simulink model "dq0inverter_DDSRF"  (R2023b)
settings: Solver=VariableStepAuto  StartTime=0.0  StopTime=10.0  RelTol=1e-3
libraries: spsSeriesRLCBranchLib x14, spsGroundLib x10, spsCurrentMeasurementLib x8, spsIGBTDiodeLib x6, slpidlib x4, spsSequenceAnalyzerLib x4, spsabctodq0Lib x4, spsVoltageMeasurementLib x4, spsBreakerLib x3, spsPLLLib x2, spsdq0toabcLib x2, spsDCVoltageSourceLib x1
settings Model: Creator=Jia Yee Wong  LastModifiedBy=Jia Yee Wong

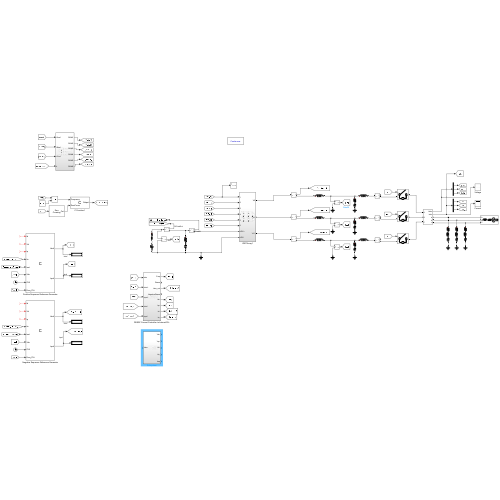
[thumbnail: Simulink's stored preview of the top-level diagram]
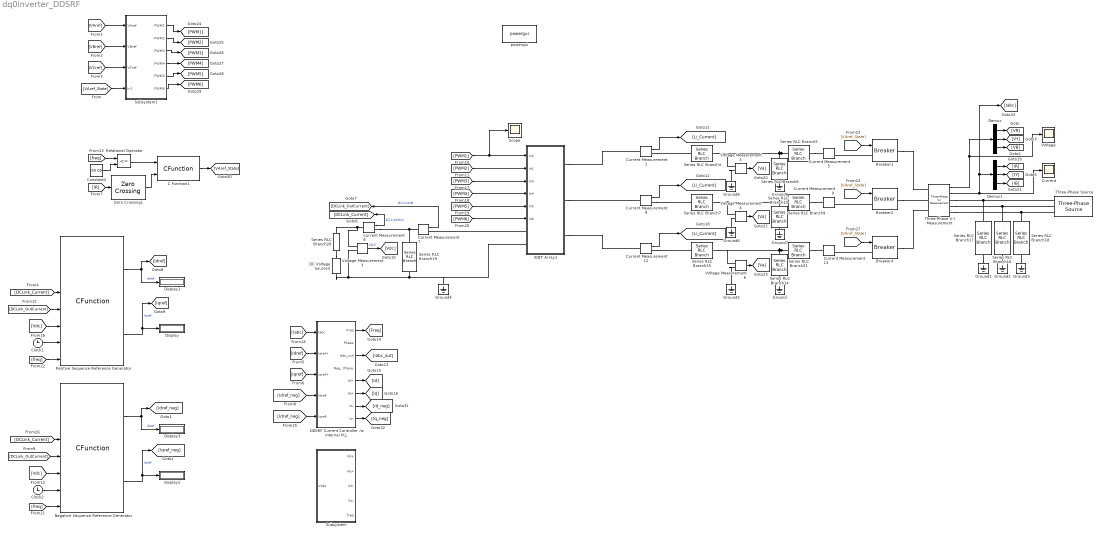
== system dq0inverter_DDSRF ==
  Breaker1 : spsBreakerLib/Breaker  InitialState=0  SwitchingTimes="[1/60  5/60]"  External=on  BreakerResistance=0.00001  SnubberResistance=30  SnubberCapacitance=47e-9  Measurements=None  MoreParameters=on  NoBreakLoop=off
  Breaker2 : spsBreakerLib/Breaker  InitialState=0  SwitchingTimes="[1/60  5/60]"  External=on  BreakerResistance=0.00001  SnubberResistance=30  SnubberCapacitance=47e-9  Measurements=None  MoreParameters=on  NoBreakLoop=off
  Breaker4 : spsBreakerLib/Breaker  InitialState=0  SwitchingTimes="[1/60  5/60]"  External=on  BreakerResistance=0.00001  SnubberResistance=30  SnubberCapacitance=47e-9  Measurements=None  MoreParameters=on  NoBreakLoop=off
  C Function1 : CFunction  OutputCode=|  SampleTime=1/50000
      | if(Frequency == true && ZeroCross == 1){
      |     Output = 1;}
      | else if(Frequency == false){
      |         Output = 0;}
  Clock1 : Clock
  Clock2 : Clock
  Constant4 : Constant  Value=50.05  SampleTime=1/50000
  Current : Scope
  Current Measurement{2,5..9,12..13} (8 alike) : spsCurrentMeasurementLib/Current Measurement  PhasorSimulation=off  OutputType=Complex  PSBequivalent=0
  DC Voltage Source3 : spsDCVoltageSourceLib/DC Voltage Source  Amplitude=400  Measurements=None
  DDSRF Current Controller /w Internal PLL : Subsystem
  Demux : Demux  Outputs=3
  Demux1 : Demux  Outputs=3
  Display{,1..3} (4 alike) : Display
  Ground{,1..9} (10 alike) : spsGroundLib/Ground  LConnTagsString=a
  IGBT Array1 : Subsystem
  Negative Sequence Reference Generator : CFunction  OutputCode=|  StartCode=|  SampleTime=1/50000
      OutputCode=|
      | if(Id!=PreviousId || Iq!=PreviousIq){
      |     if(ReferenceGenTrigger(Freq_PLL)){
      |         Idref=IdrefCalc(CLK,Vd,Iin,Iout, Vdc, Vdc);
      |   //Idref =1;
      |    Iqref=0;
      |    PreviousId=Id;
      |    PreviousIq=Iq;
      |    }
      |   
      | } else { Idref = 0; Iqref = 0;}
      StartCode=|
      | PreviousIq =0;
      | PreviousId =0;
  Positive Sequence Reference Generator : CFunction  OutputCode=|  StartCode=|  SampleTime=1/50000
      OutputCode=|
      | if(Id!=PreviousId || Iq!=PreviousIq){
      |     if(ReferenceGenTrigger(Freq_PLL)){
      |         Idref=IdrefCalc(CLK,Vd,Iin,Iout, Vdc, Vdc);
      |   //Idref =1;
      |    Iqref=0;
      |    PreviousId=Id;
      |    PreviousIq=Iq;
      |    }
      |   
      | } else { Idref = 0; Iqref = 0;}
      StartCode=|
      | PreviousIq =0;
      | PreviousId =0;
  Relational Operator : RelationalOperator  Operator=<=  OutDataTypeStr=boolean  RndMeth=Simplest  InputSameDT=off
  Scope : Scope
  Series RLC Branch10 : spsSeriesRLCBranchLib/Series RLC Branch  LConnTagsString=__new0  RConnTagsString=__new0  BranchType=RC  Resistance=120  Inductance=100e-6  SetiL0=off  InitialCurrent=0  Capacitance=5.526e-6  Setx0=off  InitialVoltage=0  Measurements=None
  Series RLC Branch14 : spsSeriesRLCBranchLib/Series RLC Branch  LConnTagsString=__new0  RConnTagsString=__new0  BranchType=RC  Resistance=120  Inductance=100e-6  SetiL0=off  InitialCurrent=0  Capacitance=5.526e-6  Setx0=off  InitialVoltage=0  Measurements=None
  Series RLC Branch15 : spsSeriesRLCBranchLib/Series RLC Branch  LConnTagsString=__new0  RConnTagsString=__new0  BranchType=L  Resistance=1  Inductance=20.4e-3  SetiL0=off  InitialCurrent=0  Capacitance=1e-6  Setx0=off  InitialVoltage=0  Measurements=None
  Series RLC Branch16 : spsSeriesRLCBranchLib/Series RLC Branch  LConnTagsString=__new0  RConnTagsString=__new0  BranchType=RLC  Resistance=1  Inductance=1e-3  SetiL0=off  InitialCurrent=0  Capacitance=1e-6  Setx0=off  InitialVoltage=0  Measurements=None
  Series RLC Branch17 : spsSeriesRLCBranchLib/Series RLC Branch  LConnTagsString=__new0  RConnTagsString=__new0  BranchType=RLC  Resistance=1  Inductance=1e-3  SetiL0=off  InitialCurrent=0  Capacitance=1e-6  Setx0=off  InitialVoltage=0  Measurements=None
  Series RLC Branch18 : spsSeriesRLCBranchLib/Series RLC Branch  LConnTagsString=__new0  RConnTagsString=__new0  BranchType=RLC  Resistance=1  Inductance=1e-3  SetiL0=off  InitialCurrent=0  Capacitance=1e-6  Setx0=off  InitialVoltage=0  Measurements=None
  Series RLC Branch19 : spsSeriesRLCBranchLib/Series RLC Branch  LConnTagsString=__new0  RConnTagsString=__new0  BranchType=RC  Resistance=1  Inductance=0  SetiL0=off  InitialCurrent=0  Capacitance=47e-3  Setx0=off  InitialVoltage=300  Measurements=None
  Series RLC Branch20 : spsSeriesRLCBranchLib/Series RLC Branch  LConnTagsString=__new0  RConnTagsString=__new0  BranchType=RL  Resistance=100  Inductance=0  SetiL0=off  InitialCurrent=0  Capacitance=1e-6  Setx0=off  InitialVoltage=0  Measurements=None
  Series RLC Branch21 : spsSeriesRLCBranchLib/Series RLC Branch  LConnTagsString=__new0  RConnTagsString=__new0  BranchType=L  Resistance=1  Inductance=148.336e-6  SetiL0=off  InitialCurrent=0  Capacitance=1e-6  Setx0=off  InitialVoltage=0  Measurements=None
  Series RLC Branch4 : spsSeriesRLCBranchLib/Series RLC Branch  LConnTagsString=__new0  RConnTagsString=__new0  BranchType=L  Resistance=1  Inductance=20.4e-3  SetiL0=off  InitialCurrent=0  Capacitance=1e-6  Setx0=off  InitialVoltage=0  Measurements=None
  Series RLC Branch5 : spsSeriesRLCBranchLib/Series RLC Branch  LConnTagsString=__new0  RConnTagsString=__new0  BranchType=L  Resistance=1  Inductance=148.336e-6  SetiL0=off  InitialCurrent=0  Capacitance=1e-6  Setx0=off  InitialVoltage=0  Measurements=None
  Series RLC Branch6 : spsSeriesRLCBranchLib/Series RLC Branch  LConnTagsString=__new0  RConnTagsString=__new0  BranchType=RC  Resistance=120  Inductance=100e-6  SetiL0=off  InitialCurrent=0  Capacitance=5.526e-6  Setx0=off  InitialVoltage=0  Measurements=None
  Series RLC Branch7 : spsSeriesRLCBranchLib/Series RLC Branch  LConnTagsString=__new0  RConnTagsString=__new0  BranchType=L  Resistance=1  Inductance=20.4e-3  SetiL0=off  InitialCurrent=0  Capacitance=1e-6  Setx0=off  InitialVoltage=0  Measurements=None
  Series RLC Branch9 : spsSeriesRLCBranchLib/Series RLC Branch  LConnTagsString=__new0  RConnTagsString=__new0  BranchType=L  Resistance=1  Inductance=148.336e-6  SetiL0=off  InitialCurrent=0  Capacitance=1e-6  Setx0=off  InitialVoltage=0  Measurements=None
  Subsystem : Subsystem
  Subsystem1 : Subsystem
  Three-Phase V-I Measurement : spsThreePhaseVIMeasurementLib/Three-Phase V-I Measurement  VoltageMeasurement=phase-to-phase  SetLabelV=off  LabelV=Vabc  Vpu=off  VpuLL=off  CurrentMeasurement=yes  SetLabelI=off  LabelI=Iabc  Ipu=off  Pbase=100e6  Vbase=500e3  OutputType=Complex  PhasorSimulation=off  PSBequivalent=0
  Three-Phase Source : spsThreePhaseSourceLib/Three-Phase Source  InternalConnection=Yg  VoltagePhases=off  Voltage=240  PhaseAngle=0  Voltage_phases=[25e3 25e3 25e3]/sqrt(3)  PhaseAngles_phases=[0 -120 +120]  Frequency=50  NonIdealSource=on  SpecifyImpedance=off  Resistance=0.001E-3  Inductance=0.001E-3  ShortCircuitLevel=100e6  BaseVoltage=240  XRratio=7  BusType=PQ  Pref=1000  Qref=0  Prefabc=[10e3, 10e3, 10e3]  Qrefabc=[0, 0, 0]  Qmin=-inf  Qmax=inf
  Voltage : Scope
  Voltage Measurement{1,3..4,6} (4 alike) : spsVoltageMeasurementLib/Voltage Measurement  PhasorSimulation=off  OutputType=Complex  PSBequivalent=0
  Zero Crossing1 : dspsigops/Zero Crossing
  powergui : spspowerguiLib/powergui  Priority=1  SimulationMode=Continuous  SampleTime=50e-6  frequency=60  Iterations=50  frequencyindice=0  Pbase=100e6  ErrMax=1e-4  UnitsV=kV  UnitsW=MW  buscounter=0  FunctionMessages=off  echomessages=off  EnableUseOfTLC=off  CurrentSourceSwitches=off  DisableSnubberDevices=off  DisableRonSwitches=off  DisableVfSwitches=off  DisplayEquations=off  AutomaticDiscreteSolvers=off  SolverType=Tustin/Backward Euler (TBE)  Interpol=off  ExternalGateDelay=off  methode=off  Ts=100  x0status=blocks  SPID=on  SwTol=0  HookPort=off  NonlinearTolerance=1e-4  nMaxIteration=100  ContinueOnMaxIteration=off  RestoreLinks=warning  ResistiveCurrentMeasurement=off  Frange=[0:2:500]  Ylog=off  Xlog=on  ShowGrid=off  save=off  variable=ZData  structure=0  ZoomFFT=off  StartTime=0.0  cycles=1  DisplayStyle=1  fundamental=60  FreqAxis=off  MaxFrequency=1000  frequencyindicesteady=1  RmsSteady=1  display=off
  wires:
  Positive Sequence Reference Generator/1 -> Display1/1, [Idref]  "Idref"
  [freq] -> Relational Operator/1
  [IR] -> Zero Crossing1/1
  Constant4/1 -> Relational Operator/2
  ? -> Positive Sequence Reference Generator/1
  Positive Sequence Reference Generator/2 -> [Iqref], Display/1  "Iqref"
  C Function1/1 -> [VAref_State]
  [DCLink_OutCurrent] -> Positive Sequence Reference Generator/5
  ? -> Positive Sequence Reference Generator/2
  Relational Operator/1 -> C Function1/1
  [Vdc] -> Positive Sequence Reference Generator/6
  Clock1/1 -> Positive Sequence Reference Generator/7
  ? -> Positive Sequence Reference Generator/3
  [freq] -> Positive Sequence Reference Generator/8
  Zero Crossing1/1 -> C Function1/2
  [DCLink_Current] -> Positive Sequence Reference Generator/4
  ? -> Negative Sequence Reference Generator/2
  [DCLink_OutCurrent] -> Negative Sequence Reference Generator/5
  Negative Sequence Reference Generator/2 -> [Iqref_neg], Display2/1  "Iqref"
  [Vdc] -> Negative Sequence Reference Generator/6
  Clock2/1 -> Negative Sequence Reference Generator/7
  [DCLink_Current] -> Negative Sequence Reference Generator/4
  [freq] -> Negative Sequence Reference Generator/8
  ? -> Negative Sequence Reference Generator/3
  ? -> Negative Sequence Reference Generator/1
  Negative Sequence Reference Generator/1 -> Display3/1, [Idref_neg]  "Idref"
  [PWM5] -> IGBT Array1/5(In5)
  Demux/1 -> [VR]
  Demux/2 -> [VY]
  [PWM3] -> IGBT Array1/3(In3)
  Demux/3 -> [VB]
  Demux1/1 -> [IR]
  [PWM4] -> IGBT Array1/4(In4)
  [PWM1] -> Scope/1, IGBT Array1/1(In2)
  [PWM6] -> IGBT Array1/6(In6)
  Three-Phase V-I Measurement/2 -> Current/1, [Iabc], Demux1/1
  Demux1/3 -> [IB]
  [PWM2] -> IGBT Array1/2(In1)
  Three-Phase V-I Measurement/1 -> Voltage/1, Demux/1
  Demux1/2 -> [IY]
  Current Measurement7/1 -> [DCLink_OutCurrent]  "DCLinkIN"
  Current Measurement6/1 -> [DCLink_Current]  "DCLinkOut"
  Voltage Measurement3/1 -> [Vdc]  "VDC"
  Current Measurement2/1 -> [Li_Current]
  [VAref_State] -> Breaker1/1
  Current Measurement8/1 -> [Li_Current]
  [VAref_State] -> Breaker2/1
  [VAref_State] -> Breaker4/1
  Current Measurement12/1 -> [Li_Current]
  Voltage Measurement1/1 -> [Va]
  Voltage Measurement4/1 -> [Va]
  Voltage Measurement6/1 -> [Va]
  Subsystem1/4(PWM4) -> [PWM4]
  Subsystem1/3(PWM3) -> [PWM3]
  Subsystem1/6(PWM6) -> [PWM6]
  [VAref] -> Subsystem1/1(VAref)
  Subsystem1/2(PWM2) -> [PWM2]
  [VBref] -> Subsystem1/2(VBref)
  Subsystem1/1(PWM1) -> [PWM1]
  [VCref] -> Subsystem1/3(VCref)
  Subsystem1/5(PWM5) -> [PWM5]
  [VAref_State] -> Subsystem1/4(In1)
  DDSRF Current Controller /w Internal PLL/3(Iabc_out) -> [Iabc_out]
  DDSRF Current Controller /w Internal PLL/1(Freq) -> [Freq]
  DDSRF Current Controller /w Internal PLL/5(Id+) -> [Id]
  DDSRF Current Controller /w Internal PLL/6(Iq+) -> [Iq]
  DDSRF Current Controller /w Internal PLL/7(Id-) -> [Id_neg]
  DDSRF Current Controller /w Internal PLL/8(Iq-) -> [Iq_neg]
  [Iabc] -> DDSRF Current Controller /w Internal PLL/1(Iabc)
  [Idref] -> DDSRF Current Controller /w Internal PLL/2(Idref+)
  [Iqref] -> DDSRF Current Controller /w Internal PLL/3(Iqref+)
  [Idref_neg] -> DDSRF Current Controller /w Internal PLL/4(Idref-)
  [Idref_neg] -> DDSRF Current Controller /w Internal PLL/5(Iqref-)
  connections:
  Three-Phase V-I Measurement/RConn3 -- Series RLC Branch18/LConn1 -- Three-Phase Source/RConn3
  Three-Phase V-I Measurement/RConn2 -- Series RLC Branch16/LConn1 -- Three-Phase Source/RConn2
  Three-Phase V-I Measurement/RConn1 -- Series RLC Branch17/LConn1 -- Three-Phase Source/RConn1
  Series RLC Branch17/RConn1 -- Ground1/LConn1
  Ground2/LConn1 -- Series RLC Branch16/RConn1
  Ground3/LConn1 -- Series RLC Branch18/RConn1
  Series RLC Branch19/RConn1 -- Ground4/LConn1 -- IGBT Array1/LConn2 -- DC Voltage Source3/LConn1 -- Voltage Measurement3/LConn2
  Series RLC Branch19/LConn1 -- Current Measurement6/RConn1 -- Current Measurement7/LConn1
  Voltage Measurement3/LConn1 -- Series RLC Branch20/LConn1 -- Current Measurement6/LConn1
  Series RLC Branch20/RConn1 -- DC Voltage Source3/RConn1
  IGBT Array1/LConn1 -- Current Measurement7/RConn1
  Series RLC Branch5/LConn1 -- Series RLC Branch6/LConn1 -- Series RLC Branch4/RConn1 -- Voltage Measurement1/LConn1
  Breaker1/RConn1 -- Three-Phase V-I Measurement/LConn1
  Series RLC Branch5/RConn1 -- Current Measurement5/LConn1
  Current Measurement2/RConn1 -- Series RLC Branch4/LConn1
  Breaker1/LConn1 -- Current Measurement5/RConn1
  Voltage Measurement4/LConn1 -- Series RLC Branch7/RConn1 -- Series RLC Branch10/LConn1 -- Series RLC Branch9/LConn1
  Current Measurement8/RConn1 -- Series RLC Branch7/LConn1
  Series RLC Branch9/RConn1 -- Current Measurement9/LConn1
  Breaker2/LConn1 -- Current Measurement9/RConn1
  Breaker2/RConn1 -- Three-Phase V-I Measurement/LConn2
  Series RLC Branch21/LConn1 -- Series RLC Branch14/LConn1 -- Series RLC Branch15/RConn1 -- Voltage Measurement6/LConn1
  Breaker4/RConn1 -- Three-Phase V-I Measurement/LConn3
  Current Measurement12/RConn1 -- Series RLC Branch15/LConn1
  Series RLC Branch21/RConn1 -- Current Measurement13/LConn1
  Breaker4/LConn1 -- Current Measurement13/RConn1
  Series RLC Branch14/RConn1 -- Ground/LConn1
  Voltage Measurement6/LConn2 -- Ground5/LConn1
  IGBT Array1/RConn2 -- Current Measurement8/LConn1
  IGBT Array1/RConn1 -- Current Measurement2/LConn1
  IGBT Array1/RConn3 -- Current Measurement12/LConn1
  Ground6/LConn1 -- Voltage Measurement4/LConn2
  Series RLC Branch10/RConn1 -- Ground7/LConn1
  Voltage Measurement1/LConn2 -- Ground8/LConn1

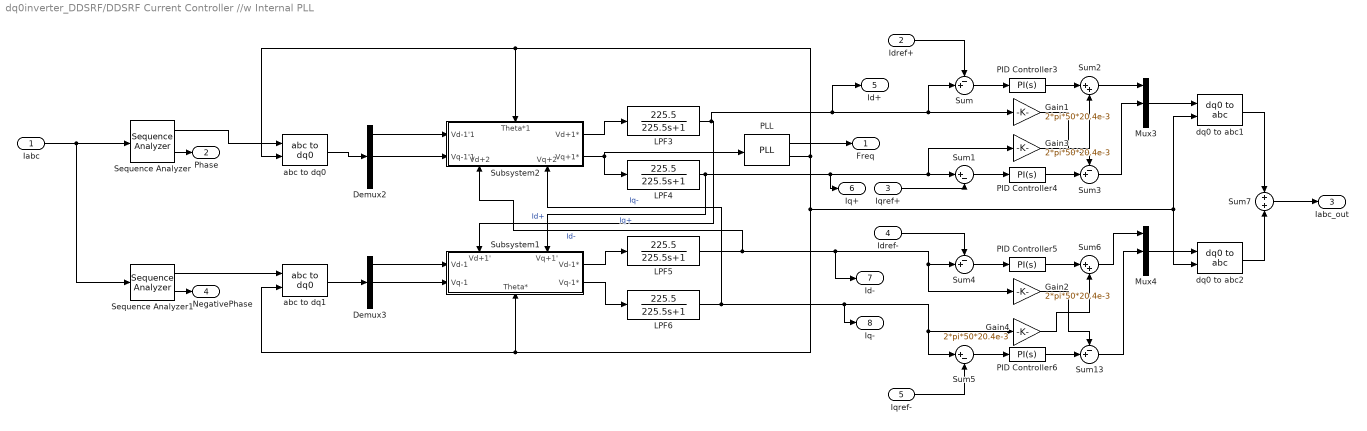
== system dq0inverter_DDSRF/DDSRF Current Controller //w Internal PLL ==
  Iabc : Inport
  Idref+ : Inport  Port=2
  Iqref+ : Inport  Port=3
  Idref- : Inport  Port=4
  Iqref- : Inport  Port=5
  Demux2 : Demux  Outputs=3
  Demux3 : Demux  Outputs=3
  Gain{1..4} (4 alike) : Gain  Gain=2*pi*50*20.4e-3
  LPF{3..6} (4 alike) : TransferFcn  Numerator=[225.5]  Denominator=[225.5 1]
  Mux3 : Mux  Inputs=3
  Mux4 : Mux  Inputs=3
  PID Controller{3..6} (4 alike) : slpidlib/PID Controller  Controller=PI  Form=Parallel  TimeDomain=Continuous-time  UseExternalTs=off  SampleTime=-1  IntegratorMethod=Forward Euler  FilterMethod=Forward Euler  ControllerParametersSource=internal  P=1  I=1  UseKiTs=off  D=0  N=100  UseFilter=on  TunerSelectOption=Transfer Function Based (PID Tuner App)  InitialConditionSource=internal  InitialConditionForIntegrator=0  InitialConditionForFilter=0  DifferentiatorICPrevScaledInput=0  ExternalReset=none  TrackingMode=off  Kt=1  LimitOutput=off  SatLimitsSource=internal  UpperSaturationLimit=inf  LowerSaturationLimit=-inf  LinearizeAsGain=on  AntiWindupMode=none  Kb=1  LimitIntegrator=off  UpperIntegratorSaturationLimit=inf  LowerIntegratorSaturationLimit=-inf  POutMin=[]  POutMax=[]  IOutMin=[]  IOutMax=[]  DOutMin=[]  DOutMax=[]  NOutMin=[]  NOutMax=[]  SumOutMin=[]  SumOutMax=[]  SaturationOutMin=[]  SaturationOutMax=[]  PParamMin=[]  PParamMax=[]  IParamMin=[]  IParamMax=[]  DParamMin=[]  DParamMax=[]  NParamMin=[]  NParamMax=[]  KbParamMin=[]  KbParamMax=[]  KtParamMin=[]  KtParamMax=[]  KbOutMin=[]  KbOutMax=[]  KtOutMin=[]  KtOutMax=[]  IntegratorOutMin=[]  IntegratorOutMax=[]  FilterOutMin=[]  FilterOutMax=[]  SumI1OutMin=[]  SumI1OutMax=[]  SumI2OutMin=[]  SumI2OutMax=[]  SumI3OutMin=[]  SumI3OutMax=[]  SumI4OutMin=[]  SumI4OutMax=[]  SumDOutMin=[]  SumDOutMax=[]  DifferentiatorOutMin=[]  DifferentiatorOutMax=[]  FilterDiffOutCoefMin=[]  FilterDiffOutCoefMax=[]  ReciprocalOutMin=[]  ReciprocalOutMax=[]  SumDenOutMin=[]  SumDenOutMax=[]  SumNumOutMin=[]  SumNumOutMax=[]  DivideOutMin=[]  DivideOutMax=[]  UdiffTsProdOutMin=[]  UdiffTsProdOutMax=[]  NTsProdOutMin=[]  NTsProdOutMax=[]  UintegralTsProdOutMin=[]  UintegralTsProdOutMax=[]  UngainTsProdOutMin=[]  UngainTsProdOutMax=[]  ClampingZeroOutDataTypeStr=Inherit: Inherit via back propagation  ClampingZeroOutMin=[]  ClampingZeroOutMax=[]  FilterDenConstantOutDataTypeStr=Inherit: Inherit via back propagation  FilterDenConstantOutMin=[]  FilterDenConstantOutMax=[]  PCopyOutDataTypeStr=Inherit: Inherit via back propagation  PCopyOutMin=[]  PCopyOutMax=[]  NCopyOutDataTypeStr=Inherit: Inherit via back propagation  NCopyOutMin=[]  NCopyOutMax=[]  IntegratorContinuousStateAttributes=''  IntegratorStateMustResolveToSignalObject=off  IntegratorRTWStateStorageClass=Auto  FilterContinuousStateAttributes=''  FilterStateMustResolveToSignalObject=off  FilterRTWStateStorageClass=Auto  ParallelPVariant=InternalParameters  IdealPVariant=Disabled  IVariant=InternalParameters  DVariant=Disabled  IntegratorVariant=Continuous  SatVariant=Disabled  AWVariant=Passthrough  PCopyVariant=Disabled  TRVariant=Disabled  FdbkBlocksVariant=Forward  IdealPFdbkVariant=Disabled  SatFdbkVariant=Disabled  DerivativeFilterVariant=Disabled  NVariant=Disabled  NCopyVariant=Disabled_SignalSpec  FilterICVariant=Disabled  IntegratorICVariant=InternalICs  ExternalResetVariant=Disabled  TRSumVariant=Passthrough  SumFdbkVariant=Disabled  SumVariant=Sum_PI  TsampFilterVariant=InternalTs  TsampNgainVariant=Passthrough  TsampIntegralVariant=Disabled_SignalSpec  ExternalSaturationOutDataTypeStr=Inherit: Same as second input
  PLL : spsPLLLib/PLL  Fmin=45  Par_Init=[0, 60]  ParK=[180, 3200, 1]  TcD=1e-4  MaxRateChangeFreq=12  FilterCutOffFreq=25  Ts=0  AGC=on
      settings: LibrarySourceBlock=sps_lib/Control/PLL
  Sequence Analyzer : spsSequenceAnalyzerLib/Sequence Analyzer  Freq=50  n=1  seq=Negative  InInit=[1, 0]  Ts=0
      settings: LibrarySourceBlock=sps_lib/Sensors and Measurements/Sequence Analyzer
  Sequence Analyzer1 : spsSequenceAnalyzerLib/Sequence Analyzer  Freq=50  n=1  seq=Negative  InInit=[1, 0]  Ts=0
      settings: LibrarySourceBlock=sps_lib/Sensors and Measurements/Sequence Analyzer
  Subsystem1 : Subsystem
      settings: PortSchema="{\"entries\":[{\"content\":{\"sides\":[{\"content\":{\"connectorIds\":[\"In1\",\"In2\"]},\"type\":\"ConnectorPlacement.EquallySpacedRectSide\",\"uuid\":\"90520742-b67b-401b-a323-e780c78b1482\"},{\"content\":{\"connectorIds\":[\"Out1\",\"Out2\"],\"side\":\"RIGHT\"},\"type\":\"ConnectorPlacement.EquallySpacedRectSide\",\"uuid\":\"13b71677-6011-49b4-a8e2-8815d9fe4fc1\"},{\"content\":{\"connectorIds\":[\"In3\",\"In4\"],\"side\":\"TOP\"},\"type\":\"ConnectorPlacement.EquallySpacedRectSide\",\"uuid\":\"b0f32480-838e-4ed7-8c04-14ce7fe710af\"},{\"content\":{\"connectorIds\":[\"In5\"],\"side\":\"BOTTOM\"},\"type\":\"ConnectorPlacement.EquallySpacedRectSide\",\"uuid\":\"11e8df11-2f01-47a5-9567-d29a5352b573\"}]},\"type\":\"ConnectorPlacement.EquallySpacedConnector\",\"uuid\":\"d99c7ffd-2341-4980-bdb2-3a875f1b77ee\"}],\"packageUris\":[\"http://schema.mathworks.com/mf0/Connector/R2020b\"],\"version\":\"1.0\"}"
  Subsystem2 : Subsystem
      settings: PortSchema="{\"entries\":[{\"content\":{\"sides\":[{\"content\":{\"connectorIds\":[\"In1\",\"In2\"]},\"type\":\"ConnectorPlacement.EquallySpacedRectSide\",\"uuid\":\"90520742-b67b-401b-a323-e780c78b1482\"},{\"content\":{\"connectorIds\":[\"Out1\",\"Out2\"],\"side\":\"RIGHT\"},\"type\":\"ConnectorPlacement.EquallySpacedRectSide\",\"uuid\":\"13b71677-6011-49b4-a8e2-8815d9fe4fc1\"},{\"content\":{\"connectorIds\":[\"In3\"],\"side\":\"TOP\"},\"type\":\"ConnectorPlacement.EquallySpacedRectSide\",\"uuid\":\"b0f32480-838e-4ed7-8c04-14ce7fe710af\"},{\"content\":{\"connectorIds\":[\"In4\",\"In5\"],\"side\":\"BOTTOM\"},\"type\":\"ConnectorPlacement.EquallySpacedRectSide\",\"uuid\":\"7441e455-6112-4477-b61e-4bb135ec9e12\"}]},\"type\":\"ConnectorPlacement.EquallySpacedConnector\",\"uuid\":\"d99c7ffd-2341-4980-bdb2-3a875f1b77ee\"}],\"packageUris\":[\"http://schema.mathworks.com/mf0/Connector/R2020b\"],\"version\":\"1.0\"}"
  Sum{,3..4,13} (4 alike) : Sum  Inputs=-+|
  Sum1 : Sum  Inputs=|+-
  Sum2 : Sum  Inputs=|++
  Sum5 : Sum  Inputs=|+-
  Sum6 : Sum  Inputs=|++
  Sum7 : Sum  Inputs=+|+
  abc to dq0 : spsabctodq0Lib/abc to dq0  Alignment=90 degrees behind phase A axis
  abc to dq1 : spsabctodq0Lib/abc to dq0  Alignment=90 degrees behind phase A axis
  dq0 to abc1 : spsdq0toabcLib/dq0 to abc  Alignment=90 degrees behind phase A axis
  dq0 to abc2 : spsdq0toabcLib/dq0 to abc  Alignment=90 degrees behind phase A axis
  Freq : Outport
  Phase : Outport  Port=2
  Iabc_out : Outport  Port=3
  NegativePhase : Outport  Port=4
  Id+ : Outport  Port=5
  Iq+ : Outport  Port=6
  Id- : Outport  Port=7
  Iq- : Outport  Port=8
  wires:
  Mux3/1 -> dq0 to abc1/1
  Demux3/1 -> Subsystem1/1(Vd-1)
  Gain2/1 -> Sum13/1
  Sum13/1 -> Mux4/2
  LPF5/1 -> Gain2/1, Sum4/2, Id-/1, Subsystem2/4(Vd+2)  "Id-"
  Sum7/1 -> Iabc_out/1
  Iabc/1 -> Sequence Analyzer1/1, Sequence Analyzer/1
  Mux4/1 -> dq0 to abc2/1
  Idref-/1 -> Sum4/1
  Sum6/1 -> Mux4/1
  LPF6/1 -> Iq-/1, Gain4/1, Sum5/1, Subsystem2/5(Vq+2)  "Iq-"
  Demux2/2 -> Subsystem2/2(Vq-1'1)
  Idref+/1 -> Sum/1
  PLL/1 -> Freq/1
  Iqref+/1 -> Sum1/2
  dq0 to abc1/1 -> Sum7/1
  LPF4/1 -> Subsystem1/4(Vq+1'), Iq+/1, Gain3/1, Sum1/1  "Iq+"
  PLL/2 -> abc to dq0/2, Subsystem2/3(Theta*1), dq0 to abc2/2, dq0 to abc1/2, abc to dq1/2, Subsystem1/5(Theta*)
  PID Controller5/1 -> Sum6/1
  Demux3/2 -> Subsystem1/2(Vq-1)
  Sum5/1 -> PID Controller6/1
  abc to dq0/1 -> Demux2/1
  Sequence Analyzer/1 -> abc to dq0/1
  Sum/1 -> PID Controller3/1
  Gain3/1 -> Sum2/2
  abc to dq1/1 -> Demux3/1
  Subsystem2/1(Vd+1*) -> LPF3/1
  Demux2/1 -> Subsystem2/1(Vd-1'1)
  Subsystem1/2(Vq-1*) -> LPF6/1
  Sum1/1 -> PID Controller4/1
  dq0 to abc2/1 -> Sum7/2
  Iqref-/1 -> Sum5/2
  Sum2/1 -> Mux3/1
  LPF3/1 -> Id+/1, Gain1/1, Sum/2, Subsystem1/3(Vd+1')  "Id+"
  Gain1/1 -> Sum3/1
  PID Controller6/1 -> Sum13/2
  Sum4/1 -> PID Controller5/1
  Sequence Analyzer1/1 -> abc to dq1/1
  Sum3/1 -> Mux3/2
  PID Controller3/1 -> Sum2/1
  Subsystem1/1(Vd-1*) -> LPF5/1
  PID Controller4/1 -> Sum3/2
  Subsystem2/2(Vq+1*) -> LPF4/1, PLL/1
  Gain4/1 -> Sum6/2
  Sequence Analyzer/2 -> Phase/1
  Sequence Analyzer1/2 -> NegativePhase/1

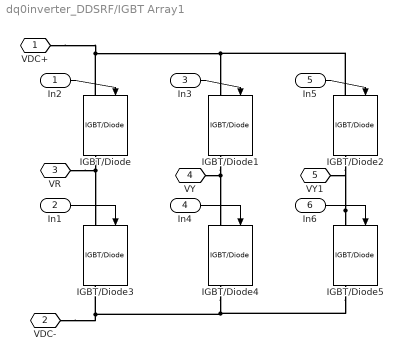
== system dq0inverter_DDSRF/IGBT Array1 ==
  In2 : Inport
  In1 : Inport  Port=2
  In3 : Inport  Port=3
  In4 : Inport  Port=4
  In5 : Inport  Port=5
  In6 : Inport  Port=6
  IGBT/Diode{,1..5} (6 alike) : spsIGBTDiodeLib/IGBT//Diode  Ron=1e-3  Rs=1e5  Cs=inf  Measurements=on
  VDC+ : PMIOPort  Side=Left
  VDC- : PMIOPort  Port=2  Side=Left
  VR : PMIOPort  Port=3  Side=Right
  VY : PMIOPort  Port=4  Side=Right
  VY1 : PMIOPort  Port=5  Side=Right
  wires:
  In1/1 -> IGBT/Diode3/1
  In4/1 -> IGBT/Diode4/1
  In3/1 -> IGBT/Diode1/1
  In2/1 -> IGBT/Diode/1
  In5/1 -> IGBT/Diode2/1
  In6/1 -> IGBT/Diode5/1
  connections:
  IGBT/Diode4/RConn1 -- IGBT/Diode5/RConn1 -- VDC-/RConn1 -- IGBT/Diode3/RConn1
  IGBT/Diode/RConn1 -- VR/RConn1 -- IGBT/Diode3/LConn1
  IGBT/Diode1/RConn1 -- VY/RConn1 -- IGBT/Diode4/LConn1
  IGBT/Diode/LConn1 -- VDC+/RConn1 -- IGBT/Diode2/LConn1 -- IGBT/Diode1/LConn1
  IGBT/Diode5/LConn1 -- IGBT/Diode2/RConn1 -- VY1/RConn1

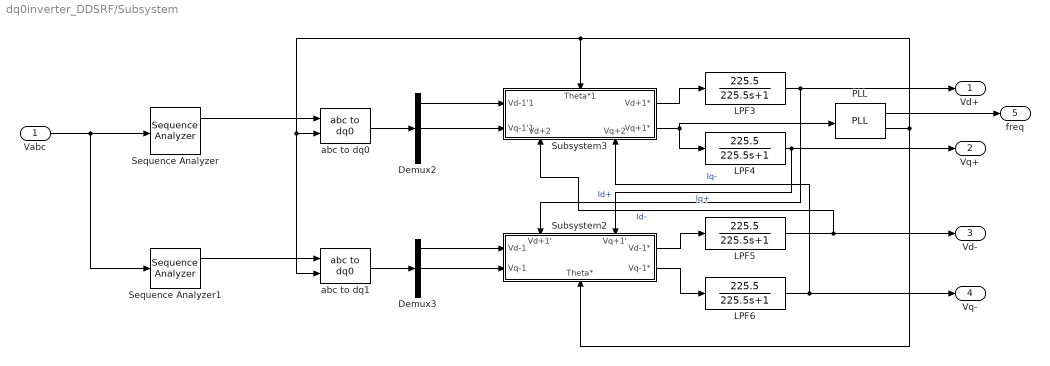
== system dq0inverter_DDSRF/Subsystem ==
  Vabc : Inport
  Demux2 : Demux  Outputs=3
  Demux3 : Demux  Outputs=3
  LPF{3..6} (4 alike) : TransferFcn  Numerator=[225.5]  Denominator=[225.5 1]
  PLL : spsPLLLib/PLL  Fmin=45  Par_Init=[0, 60]  ParK=[180, 3200, 1]  TcD=1e-4  MaxRateChangeFreq=12  FilterCutOffFreq=25  Ts=0  AGC=on
      settings: LibrarySourceBlock=sps_lib/Control/PLL
  Sequence Analyzer : spsSequenceAnalyzerLib/Sequence Analyzer  Freq=50  n=1  seq=Negative  InInit=[1, 0]  Ts=0
      settings: LibrarySourceBlock=sps_lib/Sensors and Measurements/Sequence Analyzer
  Sequence Analyzer1 : spsSequenceAnalyzerLib/Sequence Analyzer  Freq=50  n=1  seq=Negative  InInit=[1, 0]  Ts=0
      settings: LibrarySourceBlock=sps_lib/Sensors and Measurements/Sequence Analyzer
  Subsystem2 : Subsystem
      settings: PortSchema="{\"entries\":[{\"content\":{\"sides\":[{\"content\":{\"connectorIds\":[\"In1\",\"In2\"]},\"type\":\"ConnectorPlacement.EquallySpacedRectSide\",\"uuid\":\"90520742-b67b-401b-a323-e780c78b1482\"},{\"content\":{\"connectorIds\":[\"Out1\",\"Out2\"],\"side\":\"RIGHT\"},\"type\":\"ConnectorPlacement.EquallySpacedRectSide\",\"uuid\":\"13b71677-6011-49b4-a8e2-8815d9fe4fc1\"},{\"content\":{\"connectorIds\":[\"In3\",\"In4\"],\"side\":\"TOP\"},\"type\":\"ConnectorPlacement.EquallySpacedRectSide\",\"uuid\":\"b0f32480-838e-4ed7-8c04-14ce7fe710af\"},{\"content\":{\"connectorIds\":[\"In5\"],\"side\":\"BOTTOM\"},\"type\":\"ConnectorPlacement.EquallySpacedRectSide\",\"uuid\":\"11e8df11-2f01-47a5-9567-d29a5352b573\"}]},\"type\":\"ConnectorPlacement.EquallySpacedConnector\",\"uuid\":\"d99c7ffd-2341-4980-bdb2-3a875f1b77ee\"}],\"packageUris\":[\"http://schema.mathworks.com/mf0/Connector/R2020b\"],\"version\":\"1.0\"}"
  Subsystem3 : Subsystem
      settings: PortSchema="{\"entries\":[{\"content\":{\"sides\":[{\"content\":{\"connectorIds\":[\"In1\",\"In2\"]},\"type\":\"ConnectorPlacement.EquallySpacedRectSide\",\"uuid\":\"90520742-b67b-401b-a323-e780c78b1482\"},{\"content\":{\"connectorIds\":[\"Out1\",\"Out2\"],\"side\":\"RIGHT\"},\"type\":\"ConnectorPlacement.EquallySpacedRectSide\",\"uuid\":\"13b71677-6011-49b4-a8e2-8815d9fe4fc1\"},{\"content\":{\"connectorIds\":[\"In3\"],\"side\":\"TOP\"},\"type\":\"ConnectorPlacement.EquallySpacedRectSide\",\"uuid\":\"b0f32480-838e-4ed7-8c04-14ce7fe710af\"},{\"content\":{\"connectorIds\":[\"In4\",\"In5\"],\"side\":\"BOTTOM\"},\"type\":\"ConnectorPlacement.EquallySpacedRectSide\",\"uuid\":\"7441e455-6112-4477-b61e-4bb135ec9e12\"}]},\"type\":\"ConnectorPlacement.EquallySpacedConnector\",\"uuid\":\"d99c7ffd-2341-4980-bdb2-3a875f1b77ee\"}],\"packageUris\":[\"http://schema.mathworks.com/mf0/Connector/R2020b\"],\"version\":\"1.0\"}"
  abc to dq0 : spsabctodq0Lib/abc to dq0  Alignment=90 degrees behind phase A axis
  abc to dq1 : spsabctodq0Lib/abc to dq0  Alignment=90 degrees behind phase A axis
  Vd+ : Outport
  Vq+ : Outport  Port=2
  Vd- : Outport  Port=3
  Vq- : Outport  Port=4
  freq : Outport  Port=5
  wires:
  Demux2/1 -> Subsystem3/1(Vd-1'1)
  Subsystem2/1(Vd-1*) -> LPF5/1
  Vabc/1 -> Sequence Analyzer1/1, Sequence Analyzer/1
  Demux3/2 -> Subsystem2/2(Vq-1)
  Sequence Analyzer/1 -> abc to dq0/1
  Sequence Analyzer1/1 -> abc to dq1/1
  abc to dq0/1 -> Demux2/1
  LPF5/1 -> Vd-/1, Subsystem3/4(Vd+2)  "Id-"
  LPF4/1 -> Subsystem2/4(Vq+1'), Vq+/1  "Iq+"
  LPF6/1 -> Vq-/1, Subsystem3/5(Vq+2)  "Iq-"
  abc to dq1/1 -> Demux3/1
  Subsystem3/1(Vd+1*) -> LPF3/1
  Subsystem3/2(Vq+1*) -> LPF4/1, PLL/1
  Demux3/1 -> Subsystem2/1(Vd-1)
  LPF3/1 -> Vd+/1, Subsystem2/3(Vd+1')  "Id+"
  Subsystem2/2(Vq-1*) -> LPF6/1
  PLL/2 -> Subsystem2/5(Theta*), Subsystem3/3(Theta*1), abc to dq1/2, abc to dq0/2
  Demux2/2 -> Subsystem3/2(Vq-1'1)
  PLL/1 -> freq/1

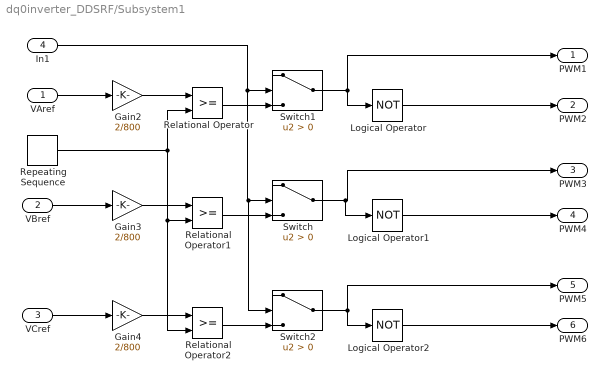
== system dq0inverter_DDSRF/Subsystem1 ==
  VAref : Inport
  VBref : Inport  Port=2
  VCref : Inport  Port=3
  In1 : Inport  Port=4
  Gain2 : Gain  Gain=2/800
  Gain3 : Gain  Gain=2/800
  Gain4 : Gain  Gain=2/800
  Logical Operator : Logic  Operator=NOT  AllPortsSameDT=off  OutDataTypeStr=boolean
  Logical Operator1 : Logic  Operator=NOT  AllPortsSameDT=off  OutDataTypeStr=boolean
  Logical Operator2 : Logic  Operator=NOT  AllPortsSameDT=off  OutDataTypeStr=boolean
  Relational Operator : RelationalOperator  OutDataTypeStr=boolean  RndMeth=Simplest  InputSameDT=off
  Relational Operator1 : RelationalOperator  OutDataTypeStr=boolean  RndMeth=Simplest  InputSameDT=off
  Relational Operator2 : RelationalOperator  OutDataTypeStr=boolean  RndMeth=Simplest  InputSameDT=off
  Repeating Sequence : simulink/Sources/Repeating Sequence  rep_seq_t=[0 0.00005 0.0001]  rep_seq_y=[-1 1 -1]
  Switch : Switch  Criteria=u2 > Threshold  SaturateOnIntegerOverflow=off  InputSameDT=off
  Switch1 : Switch  Criteria=u2 > Threshold  SaturateOnIntegerOverflow=off  InputSameDT=off
  Switch2 : Switch  Criteria=u2 > Threshold  SaturateOnIntegerOverflow=off  InputSameDT=off
  PWM1 : Outport
  PWM2 : Outport  Port=2
  PWM3 : Outport  Port=3
  PWM4 : Outport  Port=4
  PWM5 : Outport  Port=5
  PWM6 : Outport  Port=6
  wires:
  Logical Operator1/1 -> PWM4/1
  Repeating Sequence/1 -> Relational Operator/2, Relational Operator2/2, Relational Operator1/2
  VBref/1 -> Gain3/1
  Gain4/1 -> Relational Operator2/1
  VCref/1 -> Gain4/1
  Gain2/1 -> Relational Operator/1
  VAref/1 -> Gain2/1
  Gain3/1 -> Relational Operator1/1
  Logical Operator/1 -> PWM2/1
  Logical Operator2/1 -> PWM6/1
  Relational Operator2/1 -> Switch2/3
  Relational Operator1/1 -> Switch/3
  Relational Operator/1 -> Switch1/3
  In1/1 -> Switch2/2, Switch/2, Switch1/2
  Switch1/1 -> Logical Operator/1, PWM1/1
  Switch/1 -> Logical Operator1/1, PWM3/1
  Switch2/1 -> Logical Operator2/1, PWM5/1

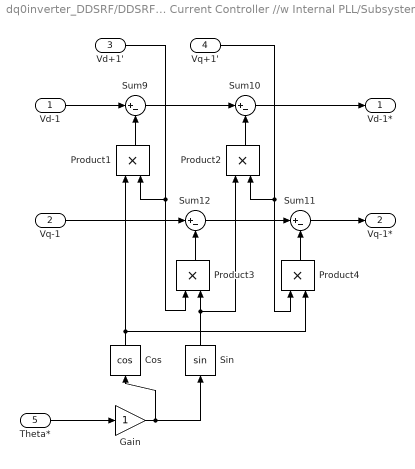
== system dq0inverter_DDSRF/DDSRF Current Controller //w Internal PLL/Subsystem1 ==
  Vd-1 : Inport
  Vq-1 : Inport  Port=2
  Vd+1' : Inport  Port=3
  Vq+1' : Inport  Port=4
  Theta* : Inport  Port=5
  Cos : Trigonometry  Operator=cos
  Gain : Gain
  Product{1..4} (4 alike) : Product
  Sin : Trigonometry
  Sum{9..12} (4 alike) : Sum  Inputs=|+-
  Vd-1* : Outport
  Vq-1* : Outport  Port=2
  wires:
  Sum11/1 -> Vq-1*/1
  Sin/1 -> Product2/1, Product3/2
  Theta*/1 -> Gain/1
  Vq+1'/1 -> Product4/1, Product2/2
  Product2/1 -> Sum10/2
  Vq-1/1 -> Sum12/1
  Sum10/1 -> Vd-1*/1
  Cos/1 -> Product4/2, Product1/1
  Sum9/1 -> Sum10/1
  Product1/1 -> Sum9/2
  Product4/1 -> Sum11/2
  Gain/1 -> Sin/1, Cos/1
  Vd+1'/1 -> Product3/1, Product1/2
  Vd-1/1 -> Sum9/1
  Product3/1 -> Sum12/2
  Sum12/1 -> Sum11/1

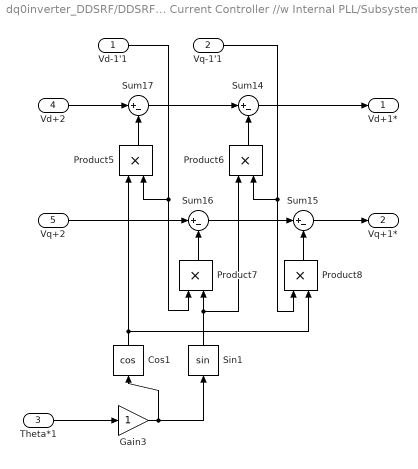
== system dq0inverter_DDSRF/DDSRF Current Controller //w Internal PLL/Subsystem2 ==
  Vd-1'1 : Inport
  Vq-1'1 : Inport  Port=2
  Theta*1 : Inport  Port=3
  Vd+2 : Inport  Port=4
  Vq+2 : Inport  Port=5
  Cos1 : Trigonometry  Operator=cos
  Gain3 : Gain
  Product{5..8} (4 alike) : Product
  Sin1 : Trigonometry
  Sum{14..17} (4 alike) : Sum  Inputs=|+-
  Vd+1* : Outport
  Vq+1* : Outport  Port=2
  wires:
  Cos1/1 -> Product8/2, Product5/1
  Vd+2/1 -> Sum17/1
  Vd-1'1/1 -> Product7/1, Product5/2
  Gain3/1 -> Sin1/1, Cos1/1
  Sin1/1 -> Product6/1, Product7/2
  Product5/1 -> Sum17/2
  Sum16/1 -> Sum15/1
  Sum14/1 -> Vd+1*/1
  Vq+2/1 -> Sum16/1
  Theta*1/1 -> Gain3/1
  Vq-1'1/1 -> Product8/1, Product6/2
  Product6/1 -> Sum14/2
  Sum17/1 -> Sum14/1
  Product8/1 -> Sum15/2
  Sum15/1 -> Vq+1*/1
  Product7/1 -> Sum16/2

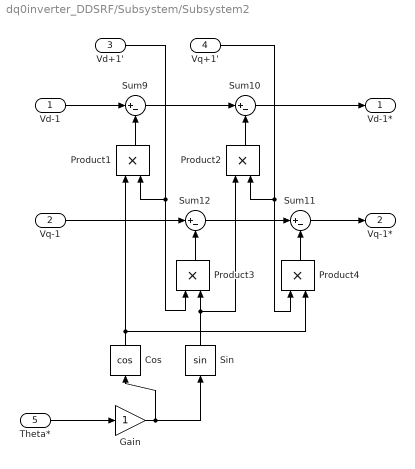
== system dq0inverter_DDSRF/Subsystem/Subsystem2 ==
  Vd-1 : Inport
  Vq-1 : Inport  Port=2
  Vd+1' : Inport  Port=3
  Vq+1' : Inport  Port=4
  Theta* : Inport  Port=5
  Cos : Trigonometry  Operator=cos
  Gain : Gain
  Product{1..4} (4 alike) : Product
  Sin : Trigonometry
  Sum{9..12} (4 alike) : Sum  Inputs=|+-
  Vd-1* : Outport
  Vq-1* : Outport  Port=2
  wires:
  Sum11/1 -> Vq-1*/1
  Sin/1 -> Product2/1, Product3/2
  Theta*/1 -> Gain/1
  Vq+1'/1 -> Product4/1, Product2/2
  Product2/1 -> Sum10/2
  Vq-1/1 -> Sum12/1
  Sum10/1 -> Vd-1*/1
  Cos/1 -> Product4/2, Product1/1
  Sum9/1 -> Sum10/1
  Product1/1 -> Sum9/2
  Product4/1 -> Sum11/2
  Gain/1 -> Sin/1, Cos/1
  Vd+1'/1 -> Product3/1, Product1/2
  Vd-1/1 -> Sum9/1
  Product3/1 -> Sum12/2
  Sum12/1 -> Sum11/1

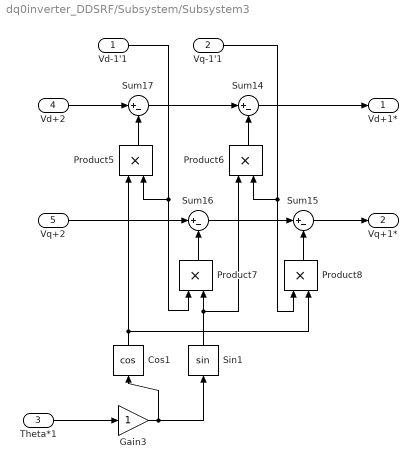
== system dq0inverter_DDSRF/Subsystem/Subsystem3 ==
  Vd-1'1 : Inport
  Vq-1'1 : Inport  Port=2
  Theta*1 : Inport  Port=3
  Vd+2 : Inport  Port=4
  Vq+2 : Inport  Port=5
  Cos1 : Trigonometry  Operator=cos
  Gain3 : Gain
  Product{5..8} (4 alike) : Product
  Sin1 : Trigonometry
  Sum{14..17} (4 alike) : Sum  Inputs=|+-
  Vd+1* : Outport
  Vq+1* : Outport  Port=2
  wires:
  Cos1/1 -> Product8/2, Product5/1
  Vd+2/1 -> Sum17/1
  Vd-1'1/1 -> Product7/1, Product5/2
  Gain3/1 -> Sin1/1, Cos1/1
  Sin1/1 -> Product6/1, Product7/2
  Product5/1 -> Sum17/2
  Sum16/1 -> Sum15/1
  Sum14/1 -> Vd+1*/1
  Vq+2/1 -> Sum16/1
  Theta*1/1 -> Gain3/1
  Vq-1'1/1 -> Product8/1, Product6/2
  Product6/1 -> Sum14/2
  Sum17/1 -> Sum14/1
  Product8/1 -> Sum15/2
  Sum15/1 -> Vq+1*/1
  Product7/1 -> Sum16/2
